simulink model "Export_H6E_Model_INL_V2_2018a"  (Simulink 9.1)
settings: Solver=VariableStepAuto  StartTime=0.0  StopTime=100  RelTol=1e-3
InitFcn:
  | Ts =2.5e-5;
  | 
  | 
  | AB_load_data;
  | AB_init;
values from neighbouring files (symbols this model uses):
  bgvmin = .8    (= 0.8)    [AB_load_data.m]
  ggv = [   0   30   40   50   60   70   80   90   95 100 ]/100    [AB_load_data.m]
  gmax = 1    [AB_load_data.m]
  gmin = 0    [AB_load_data.m]
  kd = 0.4    [AB_load_data.m]
  ki = 0.05    [AB_load_data.m]
  kp = 0.5    [AB_load_data.m]
  pgv = [ -.4 1.63 2.35 2.98 3.61 4.95 5.98 6.68 6.75 6.8 ]/8.3    [AB_load_data.m]
  pref = 1    [AB_init.m]
  rg = 0    [AB_load_data.m]
  td = 0.05    [AB_load_data.m]
  tsp = 0.05    [AB_load_data.m]
undefined symbols (not defined in the file or in its folder): s
libraries: powerlib x6, sps_avr x1
settings Model: Creator=BANEA  LastModifiedBy=BANEA
settings DataIOCC: SaveFormat=Dataset  ReturnWorkspaceOutputs=on
settings OptimizationCC: LifeSpan=auto
settings DebuggingCC: UnderspecifiedInitializationDetection=Simplified  MergeDetectMultiDrivingBlocksExec=error  SFUnexpectedBacktrackingDiag=error  SFNoUnconditionalDefaultTransitionDiag=error  SFExecutionAtInitializationDiag=warning
settings HardwareCC: ProdBitPerPointer=64  ProdBitPerSizeT=64  ProdBitPerPtrDiffT=64  ProdLargestAtomicFloat=Float  ProdIntDivRoundTo=Zero  ProdEndianess=LittleEndian  ProdWordSize=64  ProdHWDeviceType=Intel->x86-64 (Windows64)
settings ModelReferenceCC: PropagateSignalLabelsOutOfModel=on
settings SFSimCC: SimUseLocalCustomCode=on
settings RTWCC: RTWUseLocalCustomCode=on
settings CodeAppCC: StateflowObjectComments=off
settings GRTTargetCC: TargetLangStandard=C99 (ISO)  CombineOutputUpdateFcns=on  GRTInterface=off
settings ConfigComp: CovMetricSettings=dwe  CovHtmlReporting=off  CovSaveCumulativeToWorkspaceVar=off  CovSaveSingleToWorkspaceVar=off  CovExternalEMLEnable=on

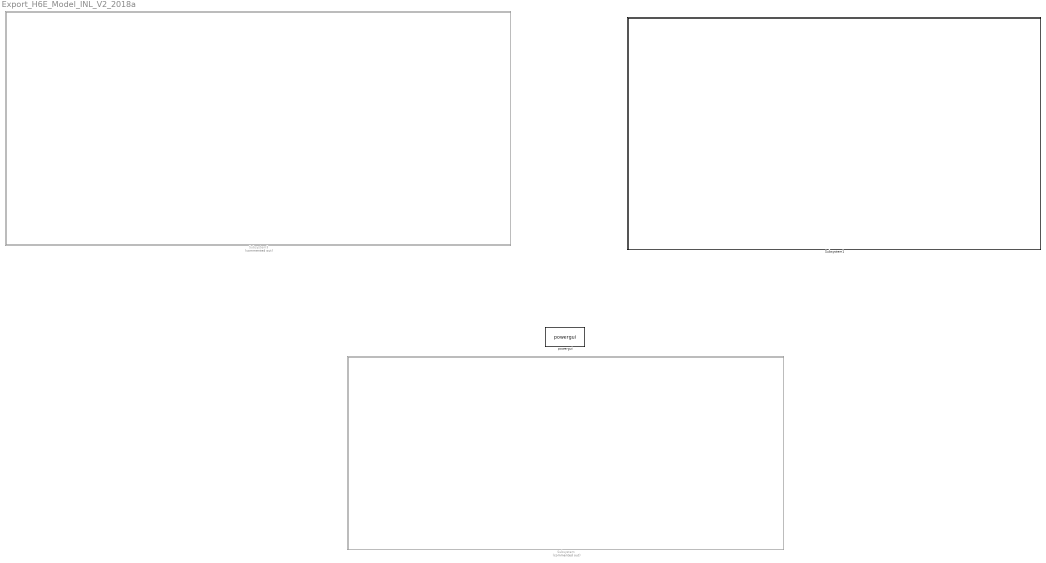
== system Export_H6E_Model_INL_V2_2018a ==
  Subsystem : Subsystem  Commented=on
  Subsystem1 : Subsystem
  Subsystem3 : Subsystem  Commented=on
  powergui : powerlib/powergui  Priority=1  SimulationMode=Discrete  SampleTime=Ts  frequency=60  Iterations=50  frequencyindice=60  Pbase=8.9e6  ErrMax=0.0001  UnitsV=kV  UnitsW=MW  buscounter=0  FunctionMessages=off  echomessages=off  EnableUseOfTLC=off  CurrentSourceSwitches=off  DisableSnubberDevices=off  DisableRonSwitches=off  DisableVfSwitches=off  DisplayEquations=off  AutomaticDiscreteSolvers=off  SolverType=Tustin/Backward Euler (TBE)  Interpol=off  ExternalGateDelay=off  methode=off  Ts=100  x0status=blocks  SPID=on  SwTol=0  HookPort=off  NonlinearTolerance=1e-4  nMaxIteration=100  ContinueOnMaxIteration=off  RestoreLinks=warning  ResistiveCurrentMeasurement=off  Frange=[0:2:500]  Ylog=off  Xlog=on  ShowGrid=off  save=off  variable=ZData  structure=0  ZoomFFT=off  StartTime=0.0  cycles=1  DisplayStyle=1  fundamental=60  FreqAxis=off  MaxFrequency=1000  frequencyindicesteady=1  RmsSteady=1  display=off

== system Export_H6E_Model_INL_V2_2018a/Subsystem ==
  note: Generator Connected Mode of
      | H6E governor turbine model
  note: Generator Connected Mode of
      | H6E governor turbine model
  note: SG Machine Connected Mode
  Governor Turbine Model : Subsystem
  "Load " : Subsystem
  Plots : Scope  NumInputPorts=4
  Scope : Scope
  Synchronous Generator Model : Subsystem
  wires:
  Governor Turbine Model/1(Pmech_p.u) -> Synchronous Generator Model/1(Pm_input (in pu))
  Synchronous Generator Model/1(<Rotor speed  wm  (pu)>) -> Governor Turbine Model/1(speed_mac)
  [speed_isol] -> Plots/3
  [gpc_isol] -> Plots/2
  [bb_isol] -> Plots/4
  [pm_isol] -> Plots/1
  [freq_gen] -> Scope/1
  connections:
  Synchronous Generator Model/RConn1 -- "Load "/LConn1
  "Load "/LConn3 -- Synchronous Generator Model/RConn3
  Synchronous Generator Model/RConn2 -- "Load "/LConn2

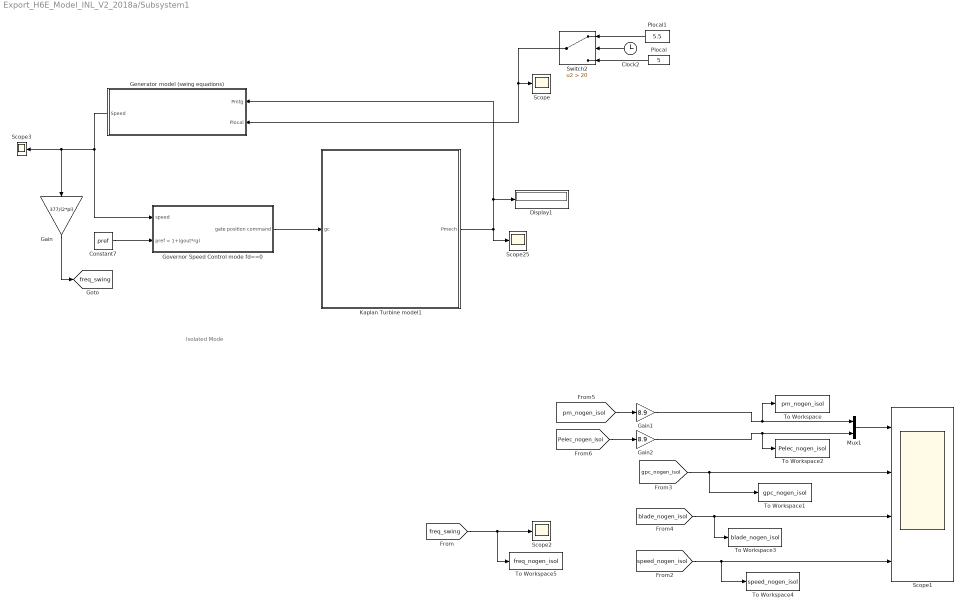
== system Export_H6E_Model_INL_V2_2018a/Subsystem1 ==
  note: Isolated Mode
  " Generator model (swing equations)" : Subsystem
  Clock2 : Clock
  Constant7 : Constant  Value=pref
  Display1 : Display
  Gain : Gain  Gain=377/(2*pi)
  Gain1 : Gain  Gain=8.9
  Gain2 : Gain  Gain=8.9
  Governor Speed Control mode fd==0 : Subsystem
  Kaplan Turbine model1 : Subsystem
  Mux1 : Mux  Inputs=2
  Plocal : Constant  Value=5
  Plocal1 : Constant  Value=5.5
  Scope{,2..3,25} (4 alike) : Scope
  Scope1 : Scope  NumInputPorts=4
  Switch2 : Switch  Criteria=u2 > Threshold  Threshold=20
  To Workspace : ToWorkspace  VariableName=pm_nogen_isol  SaveFormat=Structure With Time  SampleTime=-1
  To Workspace1 : ToWorkspace  VariableName=gpc_nogen_isol  SaveFormat=Structure With Time  SampleTime=-1
  To Workspace2 : ToWorkspace  VariableName=Pelec_nogen_isol  SaveFormat=Structure With Time  SampleTime=-1
  To Workspace3 : ToWorkspace  VariableName=blade_nogen_isol  SaveFormat=Structure With Time  SampleTime=-1
  To Workspace4 : ToWorkspace  VariableName=speed_nogen_isol  SaveFormat=Structure With Time  SampleTime=-1
  To Workspace5 : ToWorkspace  VariableName=freq_nogen_isol  SaveFormat=Structure With Time  SampleTime=-1
  tag scope: freq_swing=global
  wires:
  Clock2/1 -> Switch2/2
  Plocal1/1 -> Switch2/1
  Constant7/1 -> Governor Speed Control mode fd==0/2(pref = 1+(gout*rg))
  Kaplan Turbine model1/1(Pmech) -> Scope25/1, " Generator model (swing equations)"/1(Pmtg), Display1/1
  Plocal/1 -> Switch2/3
  Switch2/1 -> " Generator model (swing equations)"/2(Plocal), Scope/1
  Governor Speed Control mode fd==0/1("gate position command ") -> Kaplan Turbine model1/1(gc)
  " Generator model (swing equations)"/1(Speed) -> Scope3/1, Gain/1, Governor Speed Control mode fd==0/1(speed)
  Gain/1 -> [freq_swing]
  [freq_swing] -> To Workspace5/1, Scope2/1
  Mux1/1 -> Scope1/1
  [gpc_nogen_isol] -> To Workspace1/1, Scope1/2
  [blade_nogen_isol] -> To Workspace3/1, Scope1/3
  [pm_nogen_isol] -> Gain1/1
  Gain1/1 -> To Workspace/1, Mux1/1
  [Pelec_nogen_isol] -> Gain2/1
  Gain2/1 -> To Workspace2/1, Mux1/2
  [speed_nogen_isol] -> To Workspace4/1, Scope1/4

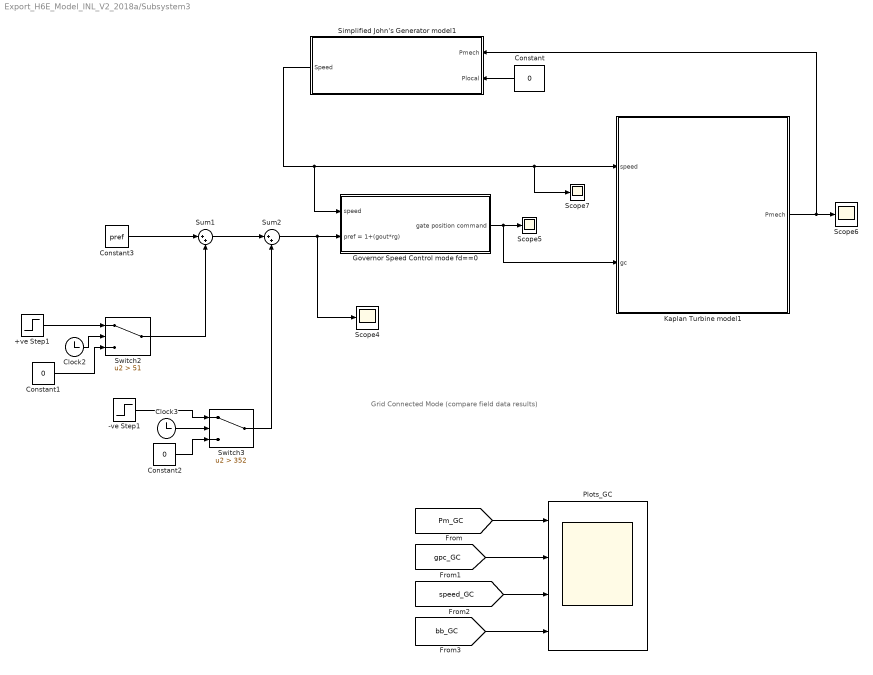
== system Export_H6E_Model_INL_V2_2018a/Subsystem3 ==
  note: Grid Connected Mode
      | (compare field data results)
  +ve Step1 : Step  Time=51  After=0.01  SampleTime=Ts
  -ve Step1 : Step  Time=352  After=-0.01  SampleTime=Ts
  Clock2 : Clock
  Clock3 : Clock
  Constant : Constant  Value=0
  Constant1 : Constant  Value=0
  Constant2 : Constant  Value=0
  Constant3 : Constant  Value=pref
  Governor Speed Control mode fd==0 : Subsystem
  Kaplan Turbine model1 : Subsystem
  Plots_GC : Scope  NumInputPorts=4
  Scope{4..7} (4 alike) : Scope
  Simplified John's Generator model1 : Subsystem
  Sum1 : Sum  Inputs=|++
  Sum2 : Sum  Inputs=|++
  Switch2 : Switch  Criteria=u2 > Threshold  Threshold=51
  Switch3 : Switch  Criteria=u2 > Threshold  Threshold=352
  wires:
  Simplified John's Generator model1/1(Speed) -> Governor Speed Control mode fd==0/1(speed), Scope7/1, Kaplan Turbine model1/1(speed)
  -ve Step1/1 -> Switch3/1
  Sum2/1 -> Scope4/1, Governor Speed Control mode fd==0/2(pref = 1+(gout*rg))
  Clock3/1 -> Switch3/2
  Constant3/1 -> Sum1/1
  Constant1/1 -> Switch2/3
  Switch2/1 -> Sum1/2
  Switch3/1 -> Sum2/2
  Sum1/1 -> Sum2/1
  Clock2/1 -> Switch2/2
  +ve Step1/1 -> Switch2/1
  Constant2/1 -> Switch3/3
  Governor Speed Control mode fd==0/1("gate position command ") -> Kaplan Turbine model1/2(gc), Scope5/1
  Kaplan Turbine model1/1(Pmech) -> Simplified John's Generator model1/1(Pmech), Scope6/1
  Constant/1 -> Simplified John's Generator model1/2(Plocal)
  [bb_GC] -> Plots_GC/4
  [Pm_GC] -> Plots_GC/1
  [speed_GC] -> Plots_GC/3
  [gpc_GC] -> Plots_GC/2

== system Export_H6E_Model_INL_V2_2018a/Subsystem/Governor Turbine Model ==
  speed_mac : Inport
  Constant5 : Constant  Value=pref
  Governor Speed Control mode (fd==0) : Subsystem
  Kaplan Turbine model : Subsystem
  Scope19 : Scope
  Pmech_p.u : Outport
  wires:
  Governor Speed Control mode (fd==0)/1("gate position command ") -> Kaplan Turbine model/2(gc), Scope19/1
  speed_mac/1 -> Kaplan Turbine model/1(speed), Governor Speed Control mode (fd==0)/1(speed)
  Constant5/1 -> Governor Speed Control mode (fd==0)/2(pref = 1+(gout*rg))
  Kaplan Turbine model/1(Pmech (in p.u.)) -> Pmech_p.u/1

== system Export_H6E_Model_INL_V2_2018a/Subsystem/Load  ==
  "  " : powerlib/Elements/Three-Phase Parallel RLC Load  LConnTagsString=A|B|C  Configuration=Y (grounded)  NominalVoltage=13.8e3  Vabc=[1e3 1e3 1e3]  Vabcp=[1e3 1e3 1e3]  NominalFrequency=60  UnbalancedPower=off  ActivePower=5e6  InductivePower=0  CapacitivePower=0  Pabc=[10e3 9e3 11e3]  QLabc=[100 90 110]  QCabc=[100 90 110]  Pabcp=[10e3 9e3 11e3]  QLabcp=[100 90 110]  QCabcp=[100 90 110]  Measurements=None  LoadType=constant Z
  0.5 MW step loading : powerlib/Elements/Three-Phase Parallel RLC Load  LConnTagsString=A|B|C  Configuration=Y (grounded)  NominalVoltage=13.8e3  Vabc=[1e3 1e3 1e3]  Vabcp=[1e3 1e3 1e3]  NominalFrequency=60  UnbalancedPower=off  ActivePower=0.5e6  InductivePower=0  CapacitivePower=0  Pabc=[10e3 9e3 11e3]  QLabc=[100 90 110]  QCabc=[100 90 110]  Pabcp=[10e3 9e3 11e3]  QLabcp=[100 90 110]  QCabcp=[100 90 110]  Measurements=None  LoadType=constant Z
  Scope15 : Scope
  Scope16 : Scope
  Three-Phase V-I Measurement2 : powerlib/Measurements/Three-Phase V-I Measurement  VoltageMeasurement=phase-to-ground  SetLabelV=off  LabelV=Vabc  Vpu=off  VpuLL=off  CurrentMeasurement=yes  SetLabelI=off  LabelI=Iabc  Ipu=off  Pbase=100e6  Vbase=500e3  OutputType=Magnitude  PhasorSimulation=off  PSBequivalent=0
  Three-Phase Breaker1 : powerlib/Elements/Three-Phase Breaker  InitialState=open  SwitchA=on  SwitchB=on  SwitchC=on  SwitchTimes=[5]  External=off  BreakerResistance=0.0001  SnubberResistance=1e10  SnubberCapacitance=inf  Measurements=None
  A : PMIOPort  Side=Left
  B : PMIOPort  Port=2  Side=Left
  C : PMIOPort  Port=3  Side=Left
  wires:
  Three-Phase V-I Measurement2/2 -> Scope16/1
  Three-Phase V-I Measurement2/1 -> Scope15/1
  connections:
  0.5 MW step loading/LConn3 -- Three-Phase Breaker1/LConn3
  Three-Phase V-I Measurement2/LConn1 -- A/RConn1
  0.5 MW step loading/LConn2 -- Three-Phase Breaker1/LConn2
  Three-Phase Breaker1/RConn2 -- Three-Phase V-I Measurement2/RConn2 -- "  "/LConn2
  0.5 MW step loading/LConn1 -- Three-Phase Breaker1/LConn1
  Three-Phase Breaker1/RConn1 -- "  "/LConn1 -- Three-Phase V-I Measurement2/RConn1
  Three-Phase V-I Measurement2/LConn2 -- B/RConn1
  Three-Phase V-I Measurement2/RConn3 -- "  "/LConn3 -- Three-Phase Breaker1/RConn3
  Three-Phase V-I Measurement2/LConn3 -- C/RConn1

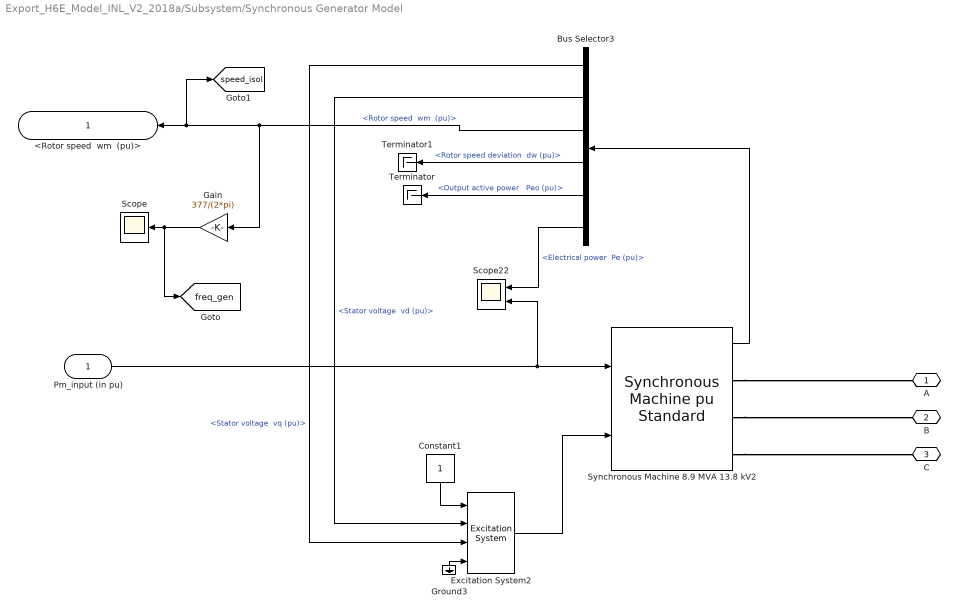
== system Export_H6E_Model_INL_V2_2018a/Subsystem/Synchronous Generator Model ==
  Pm_input (in pu) : Inport
  Bus Selector3 : BusSelector  OutputSignals="dq0 components.Stator voltage  vq (pu),dq0 components.Stator voltage  vd (pu),Mechanical.Rotor speed  wm  (pu),Mechanical.Rotor speed deviation  dw (pu),Output active power   Peo (pu),Mechanical.Electrical power  Pe (pu)"
  Constant1 : Constant
  Excitation System2 : sps_avr/Excitation System  tr=20e-3  reg=[ 300, 0.01 ]  exc=[ 1, 0 ]  tgr=[ 0, 0 ]  damp=[ 0.001, 0.1 ]  sat=[ 0, 0 ]  lim=[-2.5, 2.5, 0 ]  v0=[1,1.05779]
      settings: SourceProductBaseCode=PS
  Gain : Gain  Gain=377/(2*pi)
  Ground3 : Ground
  Scope : Scope
  Scope22 : Scope  NumInputPorts=2
  Synchronous Machine 8.9 MVA 13.8 kV2 : powerlib/Machines/Synchronous Machine pu Standard  PresetModel=No  MechanicalLoad=Mechanical power Pm  ShowDetailedParameters=on  RotorType=Salient-pole  Units=per unit standard parameters  MeasurementBus=off  NominalParameters="[ 8.9E6  13800   60 ]"  Reactances1=[ 31 32 33 34 35 36 37 ]  Reactances2=[ 1.305, 0.296, 0.252, 0.474, 0.243, 0.18 ]  dAxisTimeConstants=Short-circuit  qAxisTimeConstants=Open-circuit  TimeConstants1=[]  TimeConstants2=[]  TimeConstants3=[]  TimeConstants4=[]  TimeConstants5=[ 1.01, 0.053, 0.1 ]  TimeConstants6=[]  TimeConstants7=[]  TimeConstants8=[]  StatorResistance=2.8544e-3  Mechanical=[1.33 0 2]  PolePairs=2  InitialConditions=[0 -80.9309 0.337079 0.337079 0.337079 0 -120 120 1.05779]  SetSaturation=off  Saturation=[0.6404,0.7127,0.8441,0.9214,0.9956,1.082,1.19,1.316,1.457;0.7,0.7698,0.8872,0.9466,0.9969,1.046,1.1,1.151,1.201]  LoadFlowParameters=[2 154000000 0 0]  TsPowergui=0  TsBlock=-1  IterativeModel=Trapezoidal non iterative  IterativeDiscreteModel=Trapezoidal non iterative  BusType=swing  Pref=2e6  Qref=0  Qmin=-Inf  Qmax=Inf  PLF=0  QLF=0
      settings: AttributesFormatString=\n\n
  Terminator : Terminator
  Terminator1 : Terminator
  A : PMIOPort  Side=Right
  B : PMIOPort  Port=2  Side=Right
  C : PMIOPort  Port=3  Side=Right
  <Rotor speed  wm  (pu)> : Outport
  tag scope: freq_gen=global, speed_isol=global
  wires:
  Bus Selector3/6 -> Scope22/1  "<Electrical power  Pe (pu)>"
  Bus Selector3/2 -> Excitation System2/2  "<Stator voltage  vd (pu)>"
  Ground3/1 -> Excitation System2/4
  Bus Selector3/1 -> Excitation System2/3  "<Stator voltage  vq (pu)>"
  Excitation System2/1 -> Synchronous Machine 8.9 MVA 13.8 kV2/2
  Constant1/1 -> Excitation System2/1
  Synchronous Machine 8.9 MVA 13.8 kV2/1 -> Bus Selector3/1
  Bus Selector3/3 -> Gain/1, [speed_isol], <Rotor speed  wm  (pu)>/1  "<Rotor speed  wm  (pu)>"
  Pm_input (in pu)/1 -> Synchronous Machine 8.9 MVA 13.8 kV2/1, Scope22/2
  Bus Selector3/4 -> Terminator1/1  "<Rotor speed deviation  dw (pu)>"
  Bus Selector3/5 -> Terminator/1  "<Output active power   Peo (pu)>"
  Gain/1 -> [freq_gen], Scope/1
  connections:
  Synchronous Machine 8.9 MVA 13.8 kV2/RConn3 -- C/RConn1
  Synchronous Machine 8.9 MVA 13.8 kV2/RConn1 -- A/RConn1
  Synchronous Machine 8.9 MVA 13.8 kV2/RConn2 -- B/RConn1

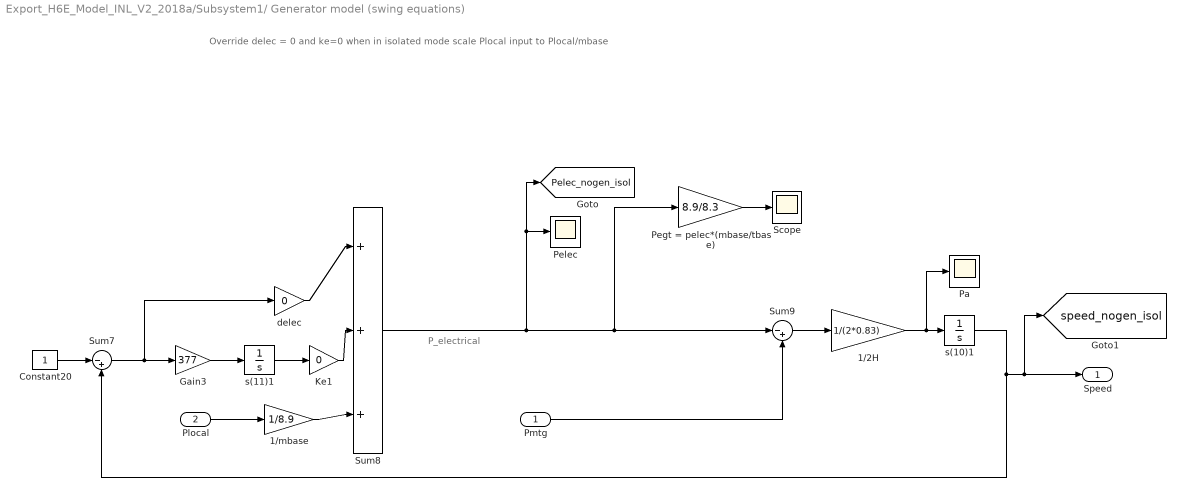
== system Export_H6E_Model_INL_V2_2018a/Subsystem1/ Generator model (swing equations) ==
  note: P_electrical
  note: Override
      | delec = 0 and ke=0
      | when in isolated mode
      | scale Plocal input to Plocal/mbase
  Pmtg : Inport
  Plocal : Inport  Port=2
  1/2H : Gain  Gain=1/(2*0.83)
  1/mbase : Gain  Gain=1/8.9
  Constant20 : Constant
  Gain3 : Gain  Gain=377
  Ke1 : Gain  Gain=0
  Pa : Scope
  Pegt = pelec*(mbase/tbase) : Gain  Gain=8.9/8.3
  Pelec : Scope
  Scope : Scope
  Sum7 : Sum  Inputs=|-+
  Sum8 : Sum  Inputs=|+++
  Sum9 : Sum  Inputs=|-+
  delec : Gain  Gain=0
  s(10)1 : Integrator  InitialCondition=s(10)
  s(11)1 : Integrator  InitialCondition=s(11)
  Speed : Outport
  tag scope: Pelec_nogen_isol=global, speed_nogen_isol=global
  wires:
  s(10)1/1 -> Sum7/2, [speed_nogen_isol], Speed/1
  Gain3/1 -> s(11)1/1
  Sum7/1 -> Gain3/1, delec/1
  Sum9/1 -> 1/2H/1
  1/2H/1 -> s(10)1/1, Pa/1
  Ke1/1 -> Sum8/2
  s(11)1/1 -> Ke1/1
  delec/1 -> Sum8/1
  Constant20/1 -> Sum7/1
  Pmtg/1 -> Sum9/2
  Plocal/1 -> 1/mbase/1
  1/mbase/1 -> Sum8/3
  Pegt = pelec*(mbase/tbase)/1 -> Scope/1
  Sum8/1 -> Sum9/1, Pegt = pelec*(mbase/tbase)/1, [Pelec_nogen_isol], Pelec/1

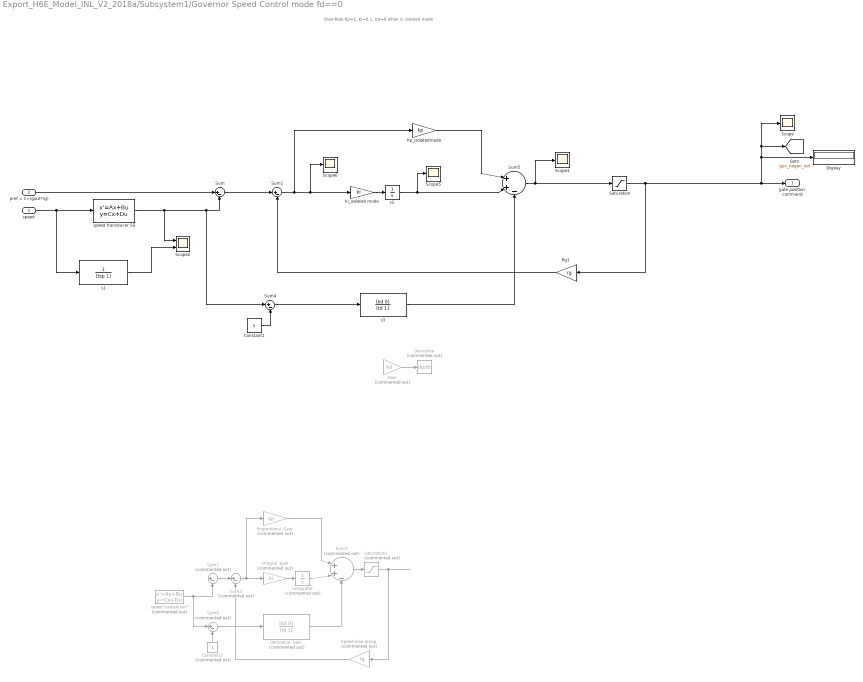
== system Export_H6E_Model_INL_V2_2018a/Subsystem1/Governor Speed Control mode fd==0 ==
  note: Over-Ride
      | Kp=1, Ki=0.1, Kd=0
      | when in isolated mode
  speed : Inport
  pref = 1+(gout*rg) : Inport  Port=2
  Constant1 : Constant
  Constant2 : Constant  Commented=on
  Derivative : Derivative  Commented=on  CoefficientInTFapproximation=td
  Derivative  Gain : TransferFcn  Commented=on  Numerator=[kd 0]  Denominator=[td 1]
  Display : Display
  Gain : Gain  Commented=on  Gain=kd
  Integral  gain : Gain  Commented=on  Gain=ki
  Integrator : Integrator  Commented=on  InitialCondition=s(2)
  Ki_isolated mode : Gain  Gain=ki
  Kp_isolatedmode : Gain  Gain=kp
  Proportional  Gain : Gain  Commented=on  Gain=kp
  Rg1 : Gain  Gain=rg
  Saturation : Saturate  UpperLimit=gmax  LowerLimit=gmin
  Saturation1 : Saturate  Commented=on  UpperLimit=gmax  LowerLimit=gmin
  Scope{,1,5..6} (4 alike) : Scope
  Scope2 : Scope  NumInputPorts=2
  Speed-load droop : Gain  Commented=on  Gain=rg
  Sum : Sum  Inputs=|+-
  Sum1 : Sum  Inputs=|+-
  Sum2 : Sum  Commented=on  Inputs=|+-
  Sum3 : Sum  Commented=on  Inputs=|+-
  Sum4 : Sum  Inputs=|+-
  Sum5 : Sum  Inputs=|++-
  Sum6 : Sum  Commented=on  Inputs=|+-
  Sum7 : Sum  Commented=on  Inputs=|++-
  s1 : TransferFcn  Denominator=[tsp 1]
  s2 : Integrator  InitialCondition=s(2)
  s3 : TransferFcn  Numerator=[kd 0]  Denominator=[td 1]
  speed transducer SS : StateSpace  A=-20  C=20  D=0  InitialCondition=s(1)/20
  speed transducer* : StateSpace  Commented=on  A=-20  C=20  D=0  InitialCondition=s(1)/20
  "gate position command " : Outport
  tag scope: gpc_nogen_isol=global
  wires:
  s1/1 -> Scope2/2
  speed/1 -> speed transducer SS/1, s1/1
  Saturation/1 -> "gate position command "/1, Display/1, [gpc_nogen_isol], Scope/1, Rg1/1
  Kp_isolatedmode/1 -> Sum5/1
  speed transducer SS/1 -> Sum4/1, Sum/2, Scope2/1
  Sum1/1 -> Kp_isolatedmode/1, Scope6/1, Ki_isolated mode/1
  Sum5/1 -> Saturation/1, Scope1/1
  pref = 1+(gout*rg)/1 -> Sum/1
  Ki_isolated mode/1 -> s2/1
  Rg1/1 -> Sum1/2
  s2/1 -> Sum5/2, Scope5/1
  Sum/1 -> Sum1/1
  s3/1 -> Sum5/3
  Sum4/1 -> s3/1
  Constant1/1 -> Sum4/2
  Gain/1 -> Derivative/1
  Constant2/1 -> Sum6/2
  Sum6/1 -> Derivative  Gain/1
  Derivative  Gain/1 -> Sum7/3
  Sum2/1 -> Sum3/1
  Integrator/1 -> Sum7/2
  Speed-load droop/1 -> Sum3/2
  Integral  gain/1 -> Integrator/1
  ? -> Sum2/1
  Sum7/1 -> Saturation1/1
  Sum3/1 -> Integral  gain/1, Proportional  Gain/1
  speed transducer*/1 -> Sum2/2, Sum6/1
  Proportional  Gain/1 -> Sum7/1
  Saturation1/1 -> Speed-load droop/1
  ? -> speed transducer*/1

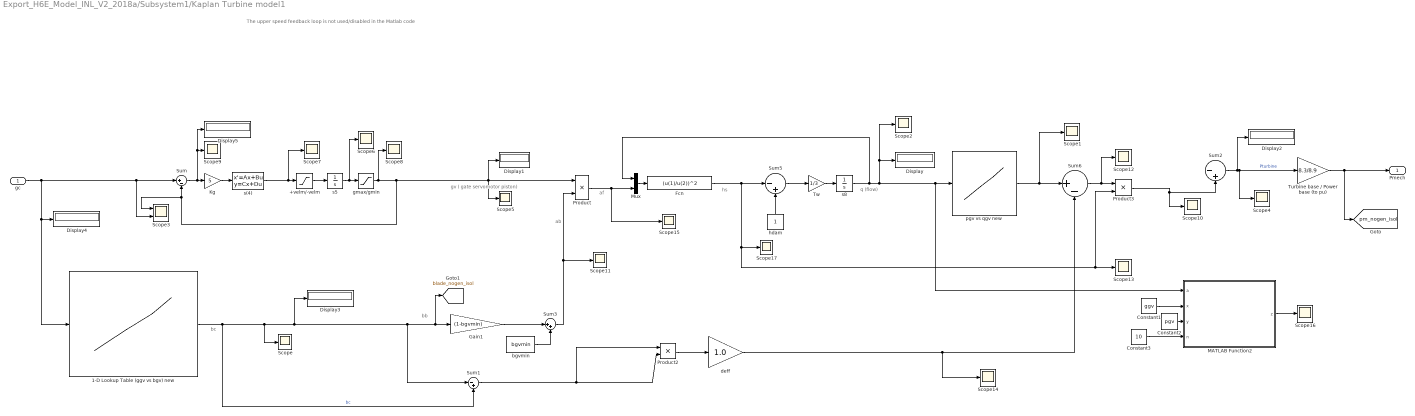
== system Export_H6E_Model_INL_V2_2018a/Subsystem1/Kaplan Turbine model1 ==
  note: bc
  note: hs
  note: q (flow)
  note: af
  note: ab
  note: gv ( gate servomotor piston)
  note: bb
  note: The upper speed feedback loop is not used/disabled in the Matlab code
  gc : Inport
  +velm/-velm : Saturate  UpperLimit=0.2  LowerLimit=-0.2
  1-D Lookup Table (ggv vs bgv) new : Lookup_n-D  NumberOfTableDimensions=1  BreakpointsForDimension1="[0\t0.300000000000000\t0.400000000000000\t0.500000000000000\t0.600000000000000\t0.700000000000000\t0.800000000000000\t0.900000000000000\t0.950000000000000\t1]"  Table="[0\t0.0950000000000000\t0.160000000000000\t0.225000000000000\t0.300000000000000\t0.535000000000000\t0.771000000000000\t0.876000000000000\t0.930000000000000\t1]"  InternalRulePriority=Speed  RndMeth=Simplest  InputSameDT=on
  Constant1 : Constant  Value=ggv
  Constant2 : Constant  Value=pgv
  Constant3 : Constant  Value=10
  Display{,1..5} (6 alike) : Display
  Fcn : Fcn  Expr=(u(1)/u(2))^2
  Gain1 : Gain  Gain=(1-bgvmin)
  Kg : Gain  Gain=5
  MATLAB Function2 : MATLAB Function  TreatAsAtomicUnit=on
  Mux : Mux  Inputs=2
  Product : Product
  Product2 : Product
  Product3 : Product
  Scope{,1..2,4..17} (17 alike) : Scope
  Scope3 : Scope  NumInputPorts=2
  Sum : Sum  Inputs=|+-
  Sum1 : Sum  Inputs=|-+
  Sum2 : Sum  Inputs=|-+
  Sum3 : Sum  Inputs=|++
  Sum5 : Sum  Inputs=|-+
  Sum6 : Sum  Inputs=|+-
  Turbine base / Power base (to pu) : Gain  Gain=8.3/8.9
  Tw : Gain  Gain=1/3
  bgvmin : Constant  Value=bgvmin
  deff : Gain  Gain=1.0
  gmax/gmin : Saturate  UpperLimit=1  LowerLimit=0
  hdam : Constant
  pgv vs qgv new : Lookup_n-D  NumberOfTableDimensions=1  BreakpointsForDimension1=[0 0.2457 0.3328 0.4225 0.5160 0.6349 0.7634 0.87777 0.9367 1.0000]  Table="[-0.0481927710843373\t0.196385542168675\t0.283132530120482\t0.359036144578313\t0.434939759036145\t0.596385542168675\t0.720481927710843\t0.804819277108434\t0.813253012048193\t0.819277108433735]"  InternalRulePriority=Speed  RndMeth=Simplest  InputSameDT=on
  s(4) : StateSpace  A=-20  C=20  D=0  InitialCondition=s(4)
  s5 : Integrator  InitialCondition=s(5)
  s8 : Integrator  InitialCondition=s(8)
  Pmech : Outport
  tag scope: blade_nogen_isol=global, pm_nogen_isol=global
  wires:
  Kg/1 -> s(4)/1
  gmax/gmin/1 -> Scope8/1, Scope5/1, Display1/1, Product/1, Sum/2, Scope3/1
  Sum2/1 -> Turbine base / Power base (to pu)/1, Scope4/1, Display2/1  "Pturbine"
  Product/1 -> Scope15/1, Mux/2
  Sum5/1 -> Tw/1
  hdam/1 -> Sum5/2
  Product3/1 -> Scope10/1, Sum2/2
  Fcn/1 -> Scope13/1, Product3/2, Scope17/1, Sum5/1
  Sum/1 -> Kg/1, Scope9/1, Display5/1
  +velm/-velm/1 -> s5/1
  s5/1 -> gmax/gmin/1, Scope6/1
  Gain1/1 -> Sum3/1
  bgvmin/1 -> Sum3/2
  pgv vs qgv new/1 -> Sum6/1, Scope1/1
  1-D Lookup Table (ggv vs bgv) new/1 -> Sum1/2, Display3/1, [blade_nogen_isol], Gain1/1, Sum1/1, Scope/1  "bc"
  gc/1 -> 1-D Lookup Table (ggv vs bgv) new/1, Display4/1, Sum/1, Scope3/2
  Sum6/1 -> Scope12/1, Product3/1
  Product2/1 -> deff/1
  deff/1 -> Scope14/1, Sum6/2
  s(4)/1 -> +velm/-velm/1, Scope7/1
  Sum3/1 -> Product/2, Scope11/1
  s8/1 -> Mux/1, MATLAB Function2/1(a), pgv vs qgv new/1, Scope2/1, Display/1
  Sum1/1 -> Product2/2, Product2/1
  Constant3/1 -> MATLAB Function2/4(n)
  Constant2/1 -> MATLAB Function2/3(y)
  Constant1/1 -> MATLAB Function2/2(x)
  MATLAB Function2/1(z) -> Scope16/1
  Mux/1 -> Fcn/1
  Tw/1 -> s8/1
  Turbine base / Power base (to pu)/1 -> [pm_nogen_isol], Pmech/1

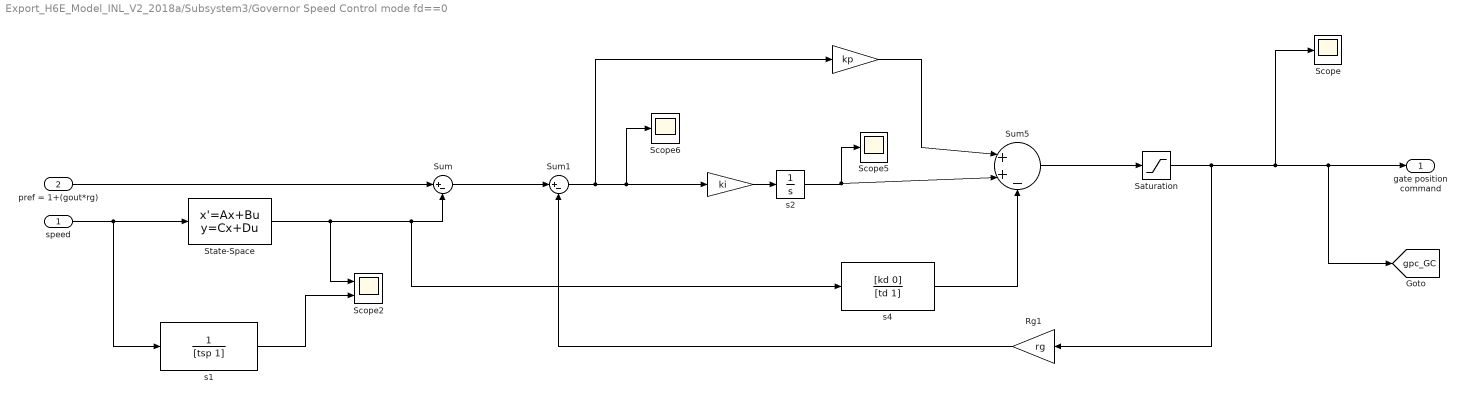
== system Export_H6E_Model_INL_V2_2018a/Subsystem3/Governor Speed Control mode fd==0 ==
  speed : Inport
  pref = 1+(gout*rg) : Inport  Port=2
  " " : Gain  Gain=kp
  "   " : Gain  Gain=ki
  Rg1 : Gain  Gain=rg
  Saturation : Saturate  UpperLimit=gmax  LowerLimit=gmin
  Scope : Scope
  Scope2 : Scope  NumInputPorts=2
  Scope5 : Scope
  Scope6 : Scope
  State-Space : StateSpace  A=-20  C=20  D=0  InitialCondition=1/20
  Sum : Sum  Inputs=|+-
  Sum1 : Sum  Inputs=|+-
  Sum5 : Sum  Inputs=|++-
  s1 : TransferFcn  Denominator=[tsp 1]
  s2 : Integrator  InitialCondition=s(2)
  s4 : TransferFcn  Numerator=[kd 0]  Denominator=[td 1]
  "gate position command " : Outport
  tag scope: gpc_GC=global
  wires:
  s1/1 -> Scope2/2
  s4/1 -> Sum5/3
  speed/1 -> State-Space/1, s1/1
  Saturation/1 -> [gpc_GC], "gate position command "/1, Scope/1, Rg1/1
  " "/1 -> Sum5/1
  State-Space/1 -> s4/1, Sum/2, Scope2/1
  Sum1/1 -> Scope6/1, "   "/1, " "/1
  Sum5/1 -> Saturation/1
  pref = 1+(gout*rg)/1 -> Sum/1
  "   "/1 -> s2/1
  Rg1/1 -> Sum1/2
  s2/1 -> Sum5/2, Scope5/1
  Sum/1 -> Sum1/1

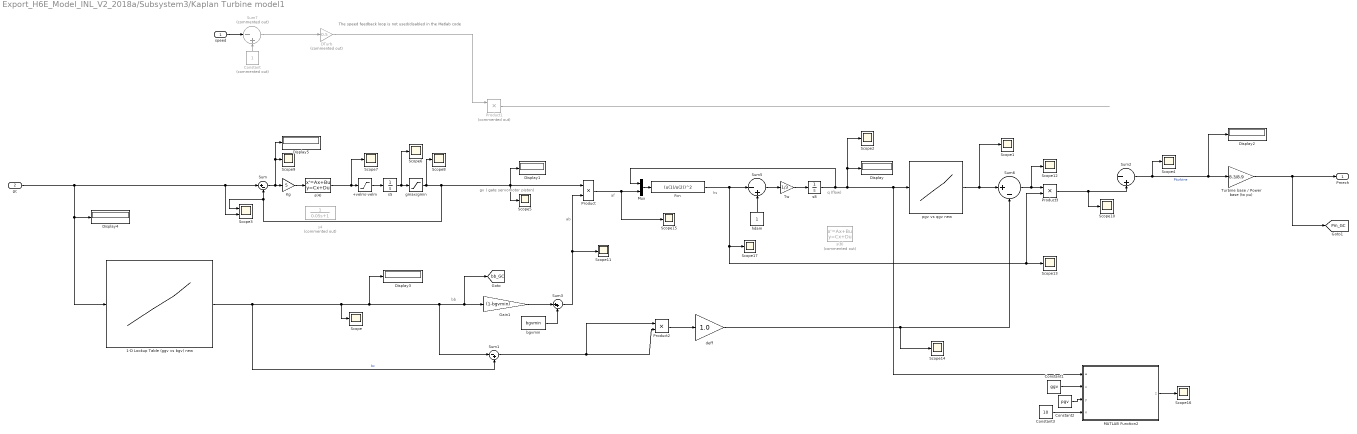
== system Export_H6E_Model_INL_V2_2018a/Subsystem3/Kaplan Turbine model1 ==
  note: hs
  note: q (flow)
  note: af
  note: ab
  note: gv ( gate servomotor piston)
  note: bb
  note: The speed feedback loop is not used/disabled in the Matlab code
  speed : Inport
  gc : Inport  Port=2
  +velm/-velm : Saturate  UpperLimit=0.2  LowerLimit=-0.2
  1-D Lookup Table (ggv vs bgv) new : Lookup_n-D  NumberOfTableDimensions=1  BreakpointsForDimension1="[0\t0.300000000000000\t0.400000000000000\t0.500000000000000\t0.600000000000000\t0.700000000000000\t0.800000000000000\t0.900000000000000\t0.950000000000000\t1]"  Table="[0\t0.0950000000000000\t0.160000000000000\t0.225000000000000\t0.300000000000000\t0.535000000000000\t0.771000000000000\t0.876000000000000\t0.930000000000000\t1]"  InternalRulePriority=Speed  RndMeth=Simplest  InputSameDT=on
  Constant : Constant  Commented=on
  Constant1 : Constant  Value=ggv
  Constant2 : Constant  Value=pgv
  Constant3 : Constant  Value=10
  DTurb : Gain  Commented=on  Gain=0.5
  Display{,1..5} (6 alike) : Display
  Fcn : Fcn  Expr=(u(1)/u(2))^2
  Gain1 : Gain  Gain=(1-bgvmin)
  Kg : Gain  Gain=5
  MATLAB Function2 : MATLAB Function  TreatAsAtomicUnit=on
  Mux : Mux  Inputs=2
  Product : Product
  Product1 : Product  Commented=on
  Product2 : Product
  Product3 : Product
  Scope{,1..2,4..17} (17 alike) : Scope
  Scope3 : Scope  NumInputPorts=2
  Sum : Sum  Inputs=|+-
  Sum1 : Sum  Inputs=|-+
  Sum2 : Sum  Inputs=|-+
  Sum3 : Sum  Inputs=|++
  Sum5 : Sum  Inputs=|-+
  Sum6 : Sum  Inputs=|+-
  Sum7 : Sum  Commented=on  Inputs=|-+
  Turbine base / Power base (to pu) : Gain  Gain=8.3/8.9
  Tw : Gain  Gain=1/3
  bgvmin : Constant  Value=bgvmin
  deff : Gain  Gain=1.0
  gmax/gmin : Saturate  UpperLimit=1  LowerLimit=0
  hdam : Constant
  pgv vs qgv new : Lookup_n-D  NumberOfTableDimensions=1  BreakpointsForDimension1=[0 0.2457 0.3328 0.4225 0.5160 0.6349 0.7634 0.87777 0.9367 1.0000]  Table="[-0.0481927710843373\t0.196385542168675\t0.283132530120482\t0.359036144578313\t0.434939759036145\t0.596385542168675\t0.720481927710843\t0.804819277108434\t0.813253012048193\t0.819277108433735]"  InternalRulePriority=Speed  RndMeth=Simplest  InputSameDT=on
  s(4) : StateSpace  A=-20  C=20  D=0  InitialCondition=0
  s(8) : StateSpace  Commented=on  A=0  C=0.3333  D=0  InitialCondition=s(8)/0.3333
  s4 : TransferFcn  Commented=on  Denominator=[0.05 1]
  s5 : Integrator  InitialCondition=s(5)
  s8 : Integrator  InitialCondition=s(8)
  Pmech : Outport
  tag scope: Pm_GC=global, bb_GC=global
  wires:
  Kg/1 -> s(4)/1
  gmax/gmin/1 -> Scope8/1, Scope5/1, Display1/1, Product/1, Sum/2, Scope3/1
  Sum2/1 -> Display2/1, Turbine base / Power base (to pu)/1, Scope4/1  "Pturbine"
  Product/1 -> Scope15/1, Mux/2
  Sum5/1 -> Tw/1
  hdam/1 -> Sum5/2
  Sum7/1 -> DTurb/1
  DTurb/1 -> Product1/1
  speed/1 -> Sum7/1
  Product3/1 -> Scope10/1, Sum2/2
  Constant/1 -> Sum7/2
  Fcn/1 -> Scope13/1, Product3/2, Scope17/1, Sum5/1
  Sum/1 -> Kg/1, Scope9/1, Display5/1
  Product1/1 -> ?
  +velm/-velm/1 -> s5/1
  s5/1 -> gmax/gmin/1, Scope6/1
  Gain1/1 -> Sum3/1
  bgvmin/1 -> Sum3/2
  pgv vs qgv new/1 -> Sum6/1, Scope1/1
  1-D Lookup Table (ggv vs bgv) new/1 -> Sum1/2, Display3/1, [bb_GC], Gain1/1, Sum1/1, Scope/1  "bc"
  gc/1 -> 1-D Lookup Table (ggv vs bgv) new/1, Display4/1, Sum/1, Scope3/2
  Sum6/1 -> Scope12/1, Product3/1
  Product2/1 -> deff/1
  deff/1 -> Scope14/1, Sum6/2
  s(4)/1 -> +velm/-velm/1, Scope7/1
  Sum3/1 -> Product/2, Scope11/1
  s8/1 -> Mux/1, MATLAB Function2/1(a), pgv vs qgv new/1, Scope2/1, Display/1
  Sum1/1 -> Product2/1, Product2/2
  Constant3/1 -> MATLAB Function2/4(n)
  Constant2/1 -> MATLAB Function2/3(y)
  Constant1/1 -> MATLAB Function2/2(x)
  MATLAB Function2/1(z) -> Scope16/1
  Mux/1 -> Fcn/1
  Tw/1 -> s8/1
  Turbine base / Power base (to pu)/1 -> [Pm_GC], Pmech/1

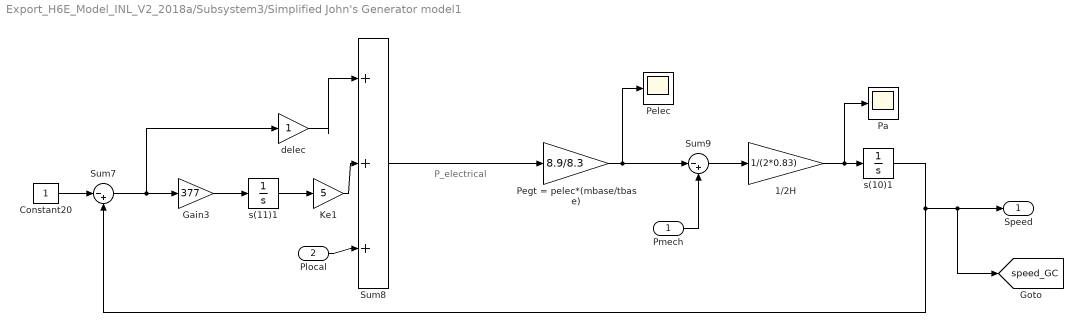
== system Export_H6E_Model_INL_V2_2018a/Subsystem3/Simplified John's Generator model1 ==
  note: P_electrical
  Pmech : Inport
  Plocal : Inport  Port=2
  1/2H : Gain  Gain=1/(2*0.83)
  Constant20 : Constant
  Gain3 : Gain  Gain=377
  Ke1 : Gain  Gain=5
  Pa : Scope
  Pegt = pelec*(mbase/tbase) : Gain  Gain=8.9/8.3
  Pelec : Scope
  Sum7 : Sum  Inputs=|-+
  Sum8 : Sum  Inputs=|+++
  Sum9 : Sum  Inputs=|-+
  delec : Gain
  s(10)1 : Integrator  InitialCondition=s(10)
  s(11)1 : Integrator  InitialCondition=s(11)
  Speed : Outport
  tag scope: speed_GC=global
  wires:
  s(10)1/1 -> Sum7/2, [speed_GC], Speed/1
  Plocal/1 -> Sum8/3
  Gain3/1 -> s(11)1/1
  Sum7/1 -> Gain3/1, delec/1
  Sum9/1 -> 1/2H/1
  1/2H/1 -> s(10)1/1, Pa/1
  Ke1/1 -> Sum8/2
  s(11)1/1 -> Ke1/1
  delec/1 -> Sum8/1
  Sum8/1 -> Pegt = pelec*(mbase/tbase)/1
  Pegt = pelec*(mbase/tbase)/1 -> Pelec/1, Sum9/1
  Constant20/1 -> Sum7/1
  Pmech/1 -> Sum9/2

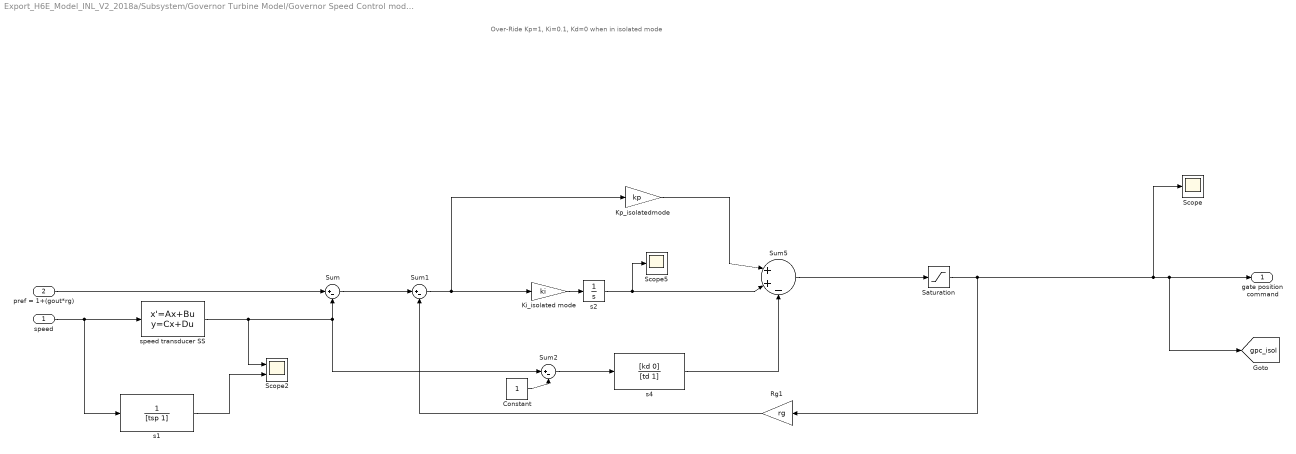
== system Export_H6E_Model_INL_V2_2018a/Subsystem/Governor Turbine Model/Governor Speed Control mode (fd==0) ==
  note: Over-Ride
      | Kp=1, Ki=0.1, Kd=0
      | when in isolated mode
  speed : Inport
  pref = 1+(gout*rg) : Inport  Port=2
  Constant : Constant
  Ki_isolated mode : Gain  Gain=ki
  Kp_isolatedmode : Gain  Gain=kp
  Rg1 : Gain  Gain=rg
  Saturation : Saturate  UpperLimit=gmax  LowerLimit=gmin
  Scope : Scope
  Scope2 : Scope  NumInputPorts=2
  Scope5 : Scope
  Sum : Sum  Inputs=|+-
  Sum1 : Sum  Inputs=|+-
  Sum2 : Sum  Inputs=|+-
  Sum5 : Sum  Inputs=|++-
  s1 : TransferFcn  Denominator=[tsp 1]
  s2 : Integrator  InitialCondition=s(2)
  s4 : TransferFcn  Numerator=[kd 0]  Denominator=[td 1]
  speed transducer SS : StateSpace  A=-20  C=20  D=0  InitialCondition=s(1)/20
  "gate position command " : Outport
  tag scope: gpc_isol=global
  wires:
  s1/1 -> Scope2/2
  s4/1 -> Sum5/3
  speed/1 -> speed transducer SS/1, s1/1
  Saturation/1 -> [gpc_isol], "gate position command "/1, Scope/1, Rg1/1
  Kp_isolatedmode/1 -> Sum5/1
  Sum1/1 -> Kp_isolatedmode/1, Ki_isolated mode/1
  Sum5/1 -> Saturation/1
  pref = 1+(gout*rg)/1 -> Sum/1
  Ki_isolated mode/1 -> s2/1
  Rg1/1 -> Sum1/2
  s2/1 -> Sum5/2, Scope5/1
  Sum/1 -> Sum1/1
  speed transducer SS/1 -> Sum2/1, Sum/2, Scope2/1
  Sum2/1 -> s4/1
  Constant/1 -> Sum2/2

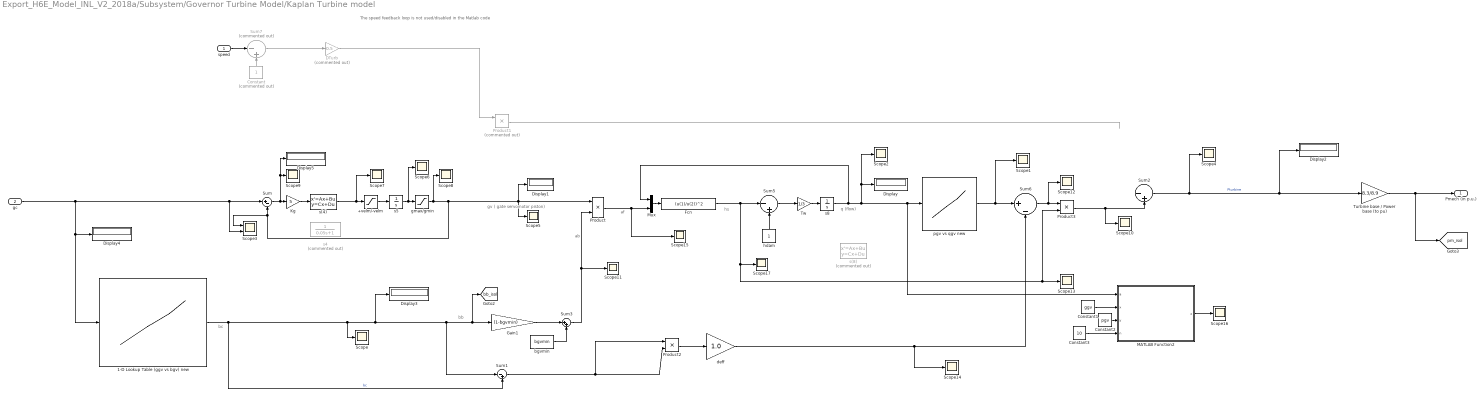
== system Export_H6E_Model_INL_V2_2018a/Subsystem/Governor Turbine Model/Kaplan Turbine model ==
  note: bc
  note: hs
  note: q (flow)
  note: af
  note: ab
  note: gv ( gate servomotor piston)
  note: bb
  note: The speed feedback loop is not used/disabled in the Matlab code
  speed : Inport
  gc : Inport  Port=2
  +velm/-velm : Saturate  UpperLimit=0.2  LowerLimit=-0.2
  1-D Lookup Table (ggv vs bgv) new : Lookup_n-D  NumberOfTableDimensions=1  BreakpointsForDimension1="[0\t0.300000000000000\t0.400000000000000\t0.500000000000000\t0.600000000000000\t0.700000000000000\t0.800000000000000\t0.900000000000000\t0.950000000000000\t1]"  Table="[0\t0.0950000000000000\t0.160000000000000\t0.225000000000000\t0.300000000000000\t0.535000000000000\t0.771000000000000\t0.876000000000000\t0.930000000000000\t1]"  InternalRulePriority=Speed  RndMeth=Simplest  InputSameDT=on
  Constant : Constant  Commented=on
  Constant1 : Constant  Value=ggv
  Constant2 : Constant  Value=pgv
  Constant3 : Constant  Value=10
  DTurb : Gain  Commented=on  Gain=0.5
  Display{,1..5} (6 alike) : Display
  Fcn : Fcn  Expr=(u(1)/u(2))^2
  Gain1 : Gain  Gain=(1-bgvmin)
  Kg : Gain  Gain=5
  MATLAB Function2 : MATLAB Function  TreatAsAtomicUnit=on
  Mux : Mux  Inputs=2
  Product : Product
  Product1 : Product  Commented=on
  Product2 : Product
  Product3 : Product
  Scope{,1..2,4..17} (17 alike) : Scope
  Scope3 : Scope  NumInputPorts=2
  Sum : Sum  Inputs=|+-
  Sum1 : Sum  Inputs=|-+
  Sum2 : Sum  Inputs=|-+
  Sum3 : Sum  Inputs=|++
  Sum5 : Sum  Inputs=|-+
  Sum6 : Sum  Inputs=|+-
  Sum7 : Sum  Commented=on  Inputs=|-+
  Turbine base / Power base (to pu) : Gain  Gain=8.3/8.9
  Tw : Gain  Gain=1/3
  bgvmin : Constant  Value=bgvmin
  deff : Gain  Gain=1.0
  gmax/gmin : Saturate  UpperLimit=1  LowerLimit=0
  hdam : Constant
  pgv vs qgv new : Lookup_n-D  NumberOfTableDimensions=1  BreakpointsForDimension1=[0 0.2457 0.3328 0.4225 0.5160 0.6349 0.7634 0.87777 0.9367 1.0000]  Table="[-0.0481927710843373\t0.196385542168675\t0.283132530120482\t0.359036144578313\t0.434939759036145\t0.596385542168675\t0.720481927710843\t0.804819277108434\t0.813253012048193\t0.819277108433735]"  InternalRulePriority=Speed  RndMeth=Simplest  InputSameDT=on
  s(4) : StateSpace  A=-20  C=20  D=0  InitialCondition=s(4)
  s(8) : StateSpace  Commented=on  A=0  C=0.3333  D=0  InitialCondition=s(8)/0.3333
  s4 : TransferFcn  Commented=on  Denominator=[0.05 1]
  s5 : Integrator  InitialCondition=s(5)
  s8 : Integrator  InitialCondition=s(8)
  Pmech (in p.u.) : Outport
  tag scope: bb_isol=global, pm_isol=global
  wires:
  Kg/1 -> s(4)/1
  gmax/gmin/1 -> Scope8/1, Scope5/1, Display1/1, Product/1, Sum/2, Scope3/1
  Sum2/1 -> Scope4/1, Display2/1, Turbine base / Power base (to pu)/1  "Pturbine"
  Product/1 -> Scope15/1, Mux/2
  Sum5/1 -> Tw/1
  hdam/1 -> Sum5/2
  Sum7/1 -> DTurb/1
  DTurb/1 -> Product1/1
  speed/1 -> Sum7/1
  Product3/1 -> Scope10/1, Sum2/2
  Constant/1 -> Sum7/2
  Fcn/1 -> Scope13/1, Product3/2, Scope17/1, Sum5/1
  Sum/1 -> Kg/1, Scope9/1, Display5/1
  Product1/1 -> ?
  +velm/-velm/1 -> s5/1
  s5/1 -> gmax/gmin/1, Scope6/1
  Gain1/1 -> Sum3/1
  bgvmin/1 -> Sum3/2
  pgv vs qgv new/1 -> Sum6/1, Scope1/1
  1-D Lookup Table (ggv vs bgv) new/1 -> Sum1/2, Display3/1, [bb_isol], Gain1/1, Sum1/1, Scope/1  "bc"
  gc/1 -> 1-D Lookup Table (ggv vs bgv) new/1, Display4/1, Sum/1, Scope3/2
  Sum6/1 -> Scope12/1, Product3/1
  Product2/1 -> deff/1
  deff/1 -> Scope14/1, Sum6/2
  s(4)/1 -> +velm/-velm/1, Scope7/1
  Sum3/1 -> Product/2, Scope11/1
  s8/1 -> Mux/1, MATLAB Function2/1(a), pgv vs qgv new/1, Scope2/1, Display/1
  Sum1/1 -> Product2/1, Product2/2
  Constant3/1 -> MATLAB Function2/4(n)
  Constant2/1 -> MATLAB Function2/3(y)
  Constant1/1 -> MATLAB Function2/2(x)
  MATLAB Function2/1(z) -> Scope16/1
  Mux/1 -> Fcn/1
  Tw/1 -> s8/1
  Turbine base / Power base (to pu)/1 -> [pm_isol], Pmech (in p.u.)/1

== matlab function Subsystem/Governor Turbine Model/Kaplan Turbine model/MATLAB Function2 ==
  data: a input double; z output double; x input double; y input double; n input double
%
% linear interpolation via table of n points 
% input is a
% independent variable is x
% dependent variable is y
% 
function z = interp( a, x, y, n)
z = 0;

if ( a >  x(n) ) z = y(n); return;  end;
if ( a <= x(1) ) z = y(1); return;  end;
for i = 1 : n-1
    if ( a <= x(i+1) )
        z = y(i) + (a-x(i))*(y(i+1)-y(i))/(x(i+1)-x(i));
        return;
    end
end
    
end

== matlab function Subsystem3/Kaplan Turbine model1/MATLAB Function2 ==
  data: a input double; z output double; x input double; y input double; n input double
%
% linear interpolation via table of n points 
% input is a
% independent variable is x
% dependent variable is y
% 
function z = interp( a, x, y, n)
z = 0;

if ( a >  x(n) ) z = y(n); return;  end;
if ( a <= x(1) ) z = y(1); return;  end;
for i = 1 : n-1
    if ( a <= x(i+1) )
        z = y(i) + (a-x(i))*(y(i+1)-y(i))/(x(i+1)-x(i));
        return;
    end
end
    
end

== matlab function Subsystem1/Kaplan Turbine model1/MATLAB Function2 ==
  data: a input double; z output double; x input double; y input double; n input double
%
% linear interpolation via table of n points 
% input is a
% independent variable is x
% dependent variable is y
% 
function z = interp( a, x, y, n)
z = 0;

if ( a >  x(n) ) z = y(n); return;  end;
if ( a <= x(1) ) z = y(1); return;  end;
for i = 1 : n-1
    if ( a <= x(i+1) )
        z = y(i) + (a-x(i))*(y(i+1)-y(i))/(x(i+1)-x(i));
        return;
    end
end
    
end
